simulink model "Wheel"  (R2018b)
settings: Solver=VariableStepAuto  StartTime=0.0  StopTime=5  RelTol=1e-3
values from neighbouring files (symbols this model uses):
  Kt = 14e4    (= 140000)    [CarQuarterParam.m]
  M2 = 20    [CarQuarterParam.m]
settings Model: Creator=Reece Bell  LastModifiedBy=Reece Bell

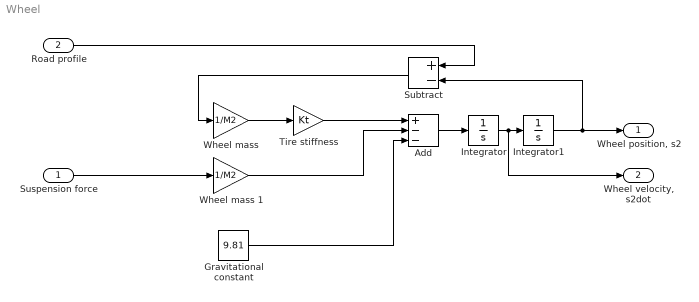
== system Wheel ==
  Suspension force : Inport
  "Road profile " : Inport  Port=2
  Add : Sum  Inputs=+--
  "Gravitational constant " : Constant  Value=9.81
  Integrator : Integrator
  Integrator1 : Integrator
  Subtract : Sum  Inputs=+-
  "Tire stiffness " : Gain  Gain=Kt
  "Wheel mass " : Gain  Gain=1/M2
  Wheel mass 1 : Gain  Gain=1/M2
  "Wheel position, s2 " : Outport
  "Wheel velocity, s2dot " : Outport  Port=2
  wires:
  "Gravitational constant "/1 -> Add/3
  Add/1 -> Integrator/1
  Integrator/1 -> "Wheel velocity, s2dot "/1, Integrator1/1
  Integrator1/1 -> Subtract/2, "Wheel position, s2 "/1
  "Tire stiffness "/1 -> Add/1
  "Road profile "/1 -> Subtract/1
  "Wheel mass "/1 -> "Tire stiffness "/1
  Subtract/1 -> "Wheel mass "/1
  Suspension force/1 -> Wheel mass 1/1
  Wheel mass 1/1 -> Add/2
